simulink model "BLDC_speedcontroller_regenbraking"  (R2017a)
settings: Solver=VariableStepAuto  StartTime=0.0  StopTime=5  MaxStep=1e-4  RelTol=1e-3
undefined symbols (not defined in the file): Ion, Lithium, Ts
libraries: powerlib x14, simulink x12, electricdrivelib x2
settings Model: Creator=Jay Anil Puranik  LastModifiedBy=Jay Anil Puranik

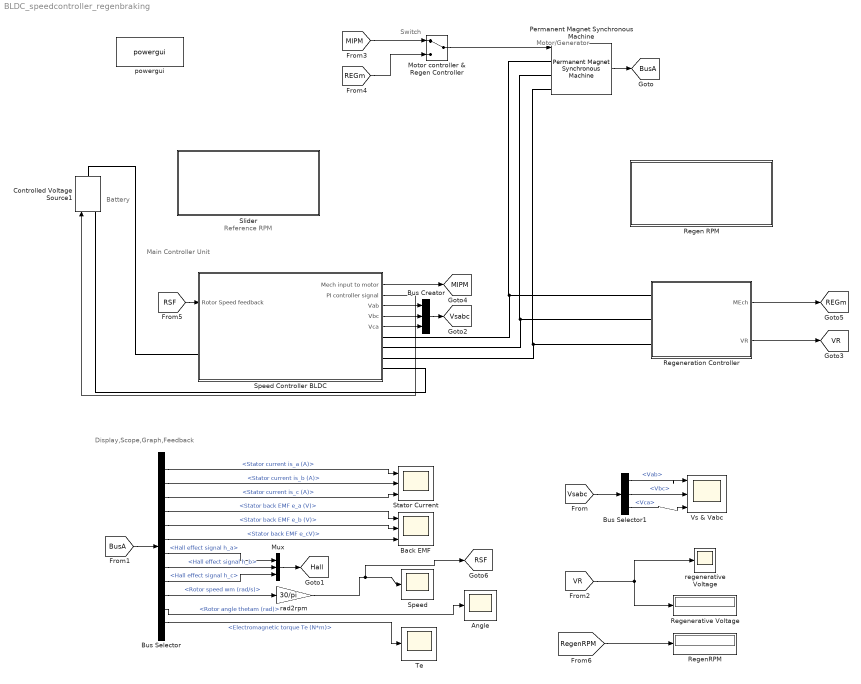
== system BLDC_speedcontroller_regenbraking ==
  note: Reference RPM
  note: Display,Scope,Graph,Feedback
  note: Main Controller Unit
  note: Motor/Generator
  note: Switch
  note: Battery
  " Angle " : Scope
  "Back EMF " : Scope  NumInputPorts=3
  Bus Creator : BusCreator  Inputs=3
  Bus Selector : BusSelector  OutputSignals=Stator current is_a (A),Stator current is_b (A),Stator current is_c (A),Stator back EMF e_a (V),Stator back EMF e_b (V),Stator back EMF e_cV),Hall effect signal h_a,Hall effect signal h_b,Hall effect signal h_c,Rotor speed wm (rad/s),Rotor angle thetam (rad),Electromagnetic torque Te (N*m)
  Bus Selector1 : BusSelector  OutputSignals=Vab,Vbc,Vca
  Controlled Voltage Source1 : powerlib/Electrical Sources/Controlled Voltage Source  Initialize=on  Source_Type=DC  Amplitude=110  Phase=0  Frequency=0  Measurements=Voltage
  "Motor controller & Regen Controller " : ManualSwitch
  Mux : Mux  Inputs=3
  Permanent Magnet Synchronous Machine : powerlib/Machines/Permanent Magnet Synchronous Machine  NbPhases=3  FluxDistribution=Trapezoidal  RotorType=Round  MechanicalLoad=Torque Tm  PresetModel=No  ShowDetailedParameters=on  MeasurementBus=off  Resistance=2.8750  Inductance=8.5e-3  dqInductances=[8.5e-3, 8.5e-3]  La=0.000835  MachineConstant=Flux linkage established by magnets (V.s)  Flux=0.175  VoltageCst=146.6077  TorqueCst=1.4  Flat=120  Mechanical=[ 0.8e-3, 1e-3 4]  PolePairs=4  InitialConditions=[0,0, 0,0]  InitialConditions5ph=[0 0 0 0 0 0]  TsPowergui=0  TsBlock=-1  RefAngle=90 degrees behind phase A axis (modified Park)
      settings: SourceProductName=Simscape Power Systems
  "Regen RPM " : Subsystem  DialogController=hmiCreateDDGDialog  IsWebBlock=on  mask(MWDashboardBlock){webBlockId=a570a540-91aa-4276-bd03-00008c0634f1, webBlockType=slider, ShowInLibBrowser=on, ShowInitialText=on, HMISrcModelName=BLDC_speedcontroller_regenbraking}
      mask prompts: webBlockId "WebBlock Id"; webBlockType "WebBlock Type"; HMISrcModelName "Source Model"
      mask help: SimulinkHMI:dialogs:SliderDialogDesc
      mask Help: helpview([docroot '/mapfiles/simulink.map'], 'hmi_slider')
      mask Display:
      | if strcmp(get_param(bdroot(gcb),'BlockDiagramType'), 'library')
      |     image([(matlabroot) '/toolbox/simulink/hmi/icons/Slider.png']);
      | end
  RegenRPM : Display
  Regeneration Controller : Subsystem
  Regenerative Voltage : Display
  Slider : Subsystem  DialogController=hmiCreateDDGDialog  IsWebBlock=on  mask(MWDashboardBlock){webBlockId=640ab695-851c-4546-9140-9b28d641b0e5, webBlockType=slider, ShowInLibBrowser=on, ShowInitialText=on, HMISrcModelName=BLDC_speedcontroller_regenbraking}
      mask prompts: webBlockId "WebBlock Id"; webBlockType "WebBlock Type"; HMISrcModelName "Source Model"
      mask help: SimulinkHMI:dialogs:SliderDialogDesc
      mask Help: helpview([docroot '/mapfiles/simulink.map'], 'hmi_slider')
      mask Display:
      | if strcmp(get_param(bdroot(gcb),'BlockDiagramType'), 'library')
      |     image([(matlabroot) '/toolbox/simulink/hmi/icons/Slider.png']);
      | end
  "Speed " : Scope
  Speed Controller BLDC : Subsystem
  "Stator Current " : Scope  NumInputPorts=3
  "Te " : Scope
  "Vs & Vabc " : Scope  NumInputPorts=3
  powergui : powerlib/powergui  Priority=2  SimulationMode=Continuous  SampleTime=Ts  frequency=60  Iterations=50  frequencyindice=0  Pbase=100e6  ErrMax=1e-4  UnitsV=kV  UnitsW=MW  buscounter=0  FunctionMessages=off  echomessages=off  EnableUseOfTLC=off  CurrentSourceSwitches=off  DisableSnubberDevices=off  DisableRonSwitches=off  DisableVfSwitches=off  DisplayEquations=off  SolverType=Tustin/Backward Euler (TBE)  Interpol=off  ExternalGateDelay=off  methode=off  Ts=100  x0status=blocks  SPID=on  SwTol=0  HookPort=off  RestoreLinks=warning  ResistiveCurrentMeasurement=off  Frange=[0:2:500]  Ylog=off  Xlog=on  ShowGrid=off  save=off  variable=ZData  structure=0  ZoomFFT=on  StartTime=0.0  cycles=1  DisplayStyle=1  fundamental=60  FreqAxis=off  MaxFrequency=1000  frequencyindicesteady=1  RmsSteady=1  display=off
  rad2rpm : Gain  Gain=30/pi
  regenerative Voltage : Scope
  tag scope: BusA=global, Hall=global, MIPM=global, REGm=global, RSF=global, VR=global, Vsabc=global
  wires:
  Bus Selector/1 -> "Stator Current "/1  "<Stator current is_a (A)>"
  Bus Selector/2 -> "Stator Current "/2  "<Stator current is_b (A)>"
  Bus Selector/3 -> "Stator Current "/3  "<Stator current is_c (A)>"
  Bus Selector/4 -> "Back EMF "/1  "<Stator back EMF e_a (V)>"
  Bus Selector/5 -> "Back EMF "/2  "<Stator back EMF e_b (V)>"
  Bus Selector/6 -> "Back EMF "/3  "<Stator back EMF e_cV)>"
  Bus Selector/7 -> Mux/1  "<Hall effect signal h_a>"
  Bus Selector/9 -> Mux/3  "<Hall effect signal h_c>"
  Bus Selector/8 -> Mux/2  "<Hall effect signal h_b>"
  Bus Selector/11 -> " Angle "/1  "<Rotor angle thetam (rad)>"
  Bus Selector/12 -> "Te "/1  "<Electromagnetic torque Te (N*m)>"
  Mux/1 -> [Hall]
  Permanent Magnet Synchronous Machine/1 -> [BusA]
  [Vsabc] -> Bus Selector1/1
  Bus Creator/1 -> [Vsabc]
  Speed Controller BLDC/3(Vab) -> Bus Creator/1
  Speed Controller BLDC/4(Vbc) -> Bus Creator/2
  Speed Controller BLDC/5(Vca) -> Bus Creator/3
  Bus Selector1/1 -> "Vs & Vabc "/1  "<Vab>"
  Bus Selector1/2 -> "Vs & Vabc "/2  "<Vbc>"
  Bus Selector1/3 -> "Vs & Vabc "/3  "<Vca>"
  [BusA] -> Bus Selector/1
  [VR] -> Regenerative Voltage/1, regenerative Voltage/1
  Speed Controller BLDC/1(Mech input to motor) -> [MIPM]
  Speed Controller BLDC/2(PI controller signal) -> Controlled Voltage Source1/1
  [MIPM] -> "Motor controller & Regen Controller "/1
  Regeneration Controller/2(VR) -> [VR]
  Regeneration Controller/1(MEch) -> [REGm]
  [REGm] -> "Motor controller & Regen Controller "/2
  [RSF] -> Speed Controller BLDC/1(Rotor Speed feedback)
  [RegenRPM] -> RegenRPM/1
  "Motor controller & Regen Controller "/1 -> Permanent Magnet Synchronous Machine/1
  Bus Selector/10 -> rad2rpm/1  "<Rotor speed wm (rad/s)>"
  rad2rpm/1 -> [RSF], "Speed "/1
  connections:
  Speed Controller BLDC/RConn1 -- Permanent Magnet Synchronous Machine/LConn1 -- Regeneration Controller/LConn1
  Speed Controller BLDC/RConn2 -- Regeneration Controller/LConn2 -- Permanent Magnet Synchronous Machine/LConn2
  Speed Controller BLDC/RConn3 -- Regeneration Controller/LConn3 -- Permanent Magnet Synchronous Machine/LConn3
  Speed Controller BLDC/LConn1 -- Controlled Voltage Source1/RConn1
  Speed Controller BLDC/RConn4 -- Controlled Voltage Source1/LConn1

== system BLDC_speedcontroller_regenbraking/Regen RPM  ==

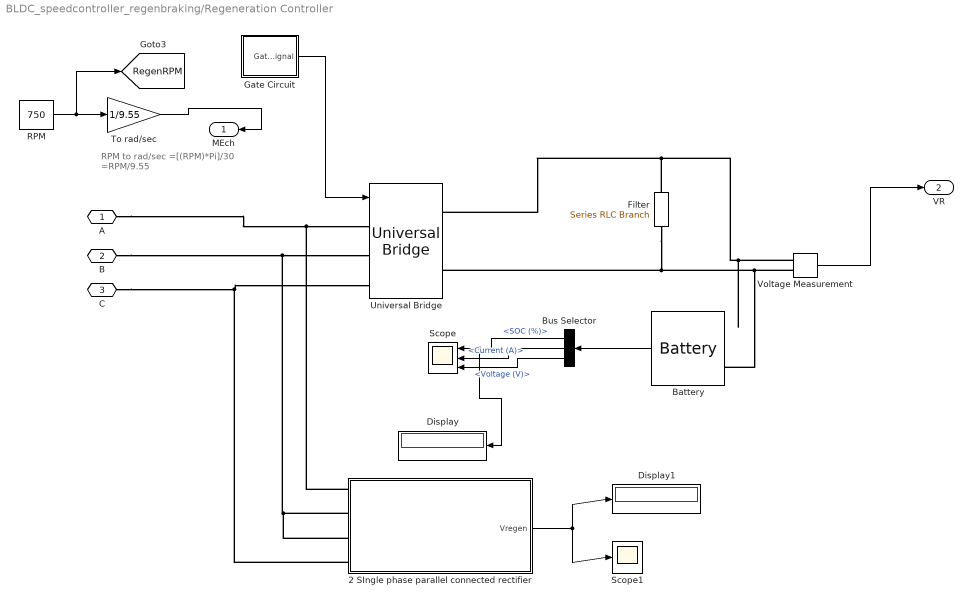
== system BLDC_speedcontroller_regenbraking/Regeneration Controller ==
  note: RPM to rad/sec
      | =[(RPM)*Pi]/30
      | =RPM/9.55
  "2 SIngle phase parallel connected rectifier " : Subsystem
  Battery : electricdrivelib/Extra Sources/Battery  BatType=Lithium-Ion  ShowTempParam=off  ThermalPreset=no  ShowAgeParam=off  NomV=7.2  NomQ=5.4  SOC=10  Batt_Tr=30  PresetModel=off  MaxQ=5.4  MinV=5.4  FullV=8.3807  Dis_rate=2.3478  R=0.013333  Normal_OP=4.8835  expZone="[7.7788      0.2653]"  current=[6.5 13 32.5]  Units=Time  Tci=20  NomT=20  T2=-30  MaxQ2=4.8  FullV2=7.1  Normal_OP2=5.655  expZone2="[6.58           1]"  Rca=0.6  ti=2000  Dp=0  Neq0=0  Tsim=1e6  Ta1=25  Qeol=5.4*0.9  Reol=0.013333*1.2  Char_age=[2.3478, 3]  Dis_age=[2.3478, 10]  N1=1500  N2=10500  N3=1000  N4=1400  Ta2=45  N5=950
  Bus Selector : BusSelector  OutputSignals=SOC (%),Current (A),Voltage (V)
  Display : Display
  Display1 : Display
  Filter : powerlib/Elements/Series RLC Branch  LConnTagsString=__new0  RConnTagsString=__new0  BranchType=C  Resistance=1  Inductance=1e-3  SetiL0=off  InitialCurrent=0  Capacitance=100e-6  Setx0=off  InitialVoltage=0  Measurements=None
  Gate Circuit : Subsystem
  "RPM " : Constant  Value=750
  Scope : Scope  NumInputPorts=3
  Scope1 : Scope
  To rad/sec : Gain  Gain=1/9.55
  Universal Bridge : powerlib/Power Electronics/Universal Bridge  Arms=3  SnubberResistance=1e5  SnubberCapacitance=inf  Device=Thyristors  Ron=1e-3  Lon=0  ForwardVoltages="[  0  0  ]"  ForwardVoltage=0  GTOparameters=[ 10e-6 , 20e-6 ]  IGBTparameters=[ 1e-6 , 2e-6 ]  Measurements=None  Measurements_2=None  converterType=Rectifier
  Voltage Measurement : powerlib/Measurements/Voltage Measurement  PhasorSimulation=off  OutputType=Magnitude  PSBequivalent=0
  A : PMIOPort  Port=1  Side=Left
  B : PMIOPort  Port=2  Side=Left
  C : PMIOPort  Port=3  Side=Left
  MEch : Outport
  VR : Outport  Port=2
  tag scope: RegenRPM=global
  wires:
  Gate Circuit/1("Gate Signal ") -> Universal Bridge/1
  Voltage Measurement/1 -> VR/1
  To rad/sec/1 -> MEch/1
  "RPM "/1 -> [RegenRPM], To rad/sec/1
  Battery/1 -> Bus Selector/1
  Bus Selector/1 -> Display/1, Scope/1  "<SOC (%)>"
  Bus Selector/2 -> Scope/2  "<Current (A)>"
  Bus Selector/3 -> Scope/3  "<Voltage (V)>"
  "2 SIngle phase parallel connected rectifier "/1("Vregen ") -> Display1/1, Scope1/1
  connections:
  B/RConn1 -- "2 SIngle phase parallel connected rectifier "/LConn3 -- "2 SIngle phase parallel connected rectifier "/LConn2 -- Universal Bridge/LConn2
  A/RConn1 -- "2 SIngle phase parallel connected rectifier "/LConn1 -- Universal Bridge/LConn1
  C/RConn1 -- "2 SIngle phase parallel connected rectifier "/LConn4 -- Universal Bridge/LConn3
  Voltage Measurement/LConn2 -- Battery/LConn2 -- Universal Bridge/RConn2 -- Filter/RConn1
  Voltage Measurement/LConn1 -- Filter/LConn1 -- Universal Bridge/RConn1

== system BLDC_speedcontroller_regenbraking/Slider ==

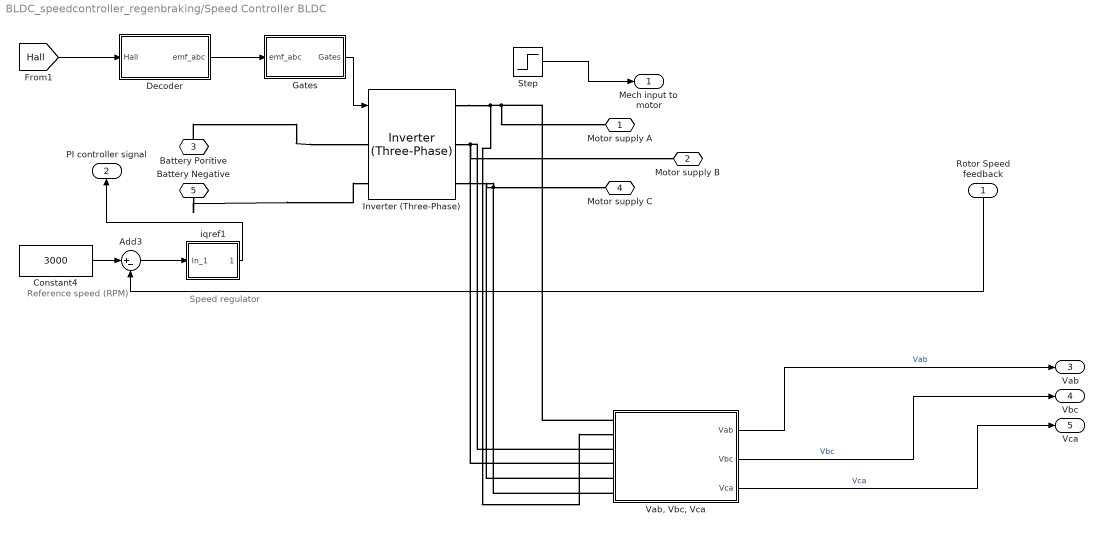
== system BLDC_speedcontroller_regenbraking/Speed Controller BLDC ==
  note: Speed
      | regulator
  note: Reference
      | speed (RPM)
  Rotor Speed feedback : Inport
  Add3 : Sum  Inputs=|+-
  Constant4 : Constant  Value=3000
  Decoder : Subsystem
  Gates : Subsystem
  Inverter (Three-Phase) : electricdrivelib/Fundamental Drive Blocks/Inverter (Three-Phase)  OverrideUsingVariant=Detailed  detailLevel=Detailed  driveType=Field-oriented control  Ts=2e-6  SnubberResistance=500  SnubberCapacitance=inf  Device=IGBT / Diodes  Ron=1  ForwardVoltages=[1.2,1.2]  GTOparameters=[1e-6,2e-6]  IGBTparameters=[1e-6,2e-6]  Measurements=All voltages and currents  converterType=Inverter  SourceFrequency=0  ReferenceFrame=Rotor  dqInductances=[8.5e-3,8.5e-3]  Inductance=8.5e-3  Ls=0  Resistance=0.2  Flux=0  Stator_sm=[2.01e-3,4.289e-4,4.477e-3,1.354e-3]  Stator_im=[14.85e-3,0.3027e-3]  Rotor=[9.295e-3,0.3027e-3]  Lm=10.46e-3  p=4
      settings: AttributesFormatString=%<BlockChoice>  SourceProductName=Simscape Power Systems  SourceProductBaseCode=PS
  Step : Step  Time=.1  After=3  SampleTime=0
  "Vab, Vbc, Vca" : Subsystem
  iqref1 : Subsystem  mask(PI Controller){I=16.61, P=.013, sat=[-100, 100]}
      mask prompts: I "Integral"; P "Proportional:"; sat "Minimum and maximum outputs:"
      mask init:
      | min=sat(1);max=sat(2);
      mask Display: disp('PI')
  Motor supply A : PMIOPort  Port=1  Side=Right
  Motor supply B : PMIOPort  Port=2  Side=Right
  "Battery Poritive " : PMIOPort  Port=3  Side=Left
  Motor supply C : PMIOPort  Port=4  Side=Right
  Battery Negative : PMIOPort  Port=5  Side=Right
  Mech input to motor : Outport
  PI controller signal : Outport  Port=2
  Vab : Outport  Port=3
  Vbc : Outport  Port=4
  Vca : Outport  Port=5
  wires:
  Rotor Speed feedback/1 -> Add3/2
  [Hall] -> Decoder/1("Hall ")
  Step/1 -> Mech input to motor/1
  Gates/1(Gates) -> Inverter (Three-Phase)/1
  Add3/1 -> iqref1/1(In_1)
  Constant4/1 -> Add3/1
  Decoder/1(emf_abc) -> Gates/1("emf_abc ")
  "Vab, Vbc, Vca"/3("Vca ") -> Vca/1  "Vca"
  "Vab, Vbc, Vca"/1("Vab ") -> Vab/1  "Vab"
  "Vab, Vbc, Vca"/2("Vbc ") -> Vbc/1  "Vbc"
  iqref1/1(Out_1) -> PI controller signal/1
  connections:
  "Vab, Vbc, Vca"/LConn1 -- Inverter (Three-Phase)/RConn1 -- "Vab, Vbc, Vca"/LConn2 -- Motor supply A/RConn1
  Battery Negative/RConn1 -- Inverter (Three-Phase)/LConn2
  "Battery Poritive "/RConn1 -- Inverter (Three-Phase)/LConn1
  Inverter (Three-Phase)/RConn2 -- "Vab, Vbc, Vca"/LConn3 -- Motor supply B/RConn1 -- "Vab, Vbc, Vca"/LConn4
  "Vab, Vbc, Vca"/LConn6 -- "Vab, Vbc, Vca"/LConn5 -- Inverter (Three-Phase)/RConn3 -- Motor supply C/RConn1

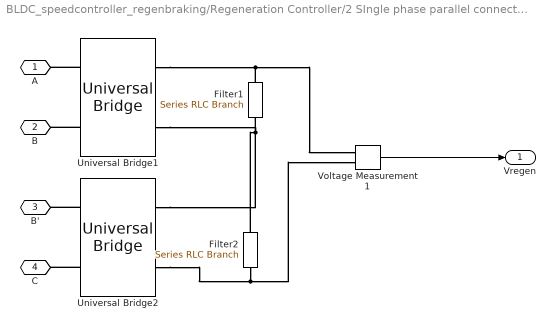
== system BLDC_speedcontroller_regenbraking/Regeneration Controller/2 SIngle phase parallel connected rectifier  ==
  Filter1 : powerlib/Elements/Series RLC Branch  LConnTagsString=__new0  RConnTagsString=__new0  BranchType=C  Resistance=1  Inductance=1e-3  SetiL0=off  InitialCurrent=0  Capacitance=100e-6  Setx0=off  InitialVoltage=0  Measurements=None
  Filter2 : powerlib/Elements/Series RLC Branch  LConnTagsString=__new0  RConnTagsString=__new0  BranchType=C  Resistance=1  Inductance=1e-3  SetiL0=off  InitialCurrent=0  Capacitance=100e-6  Setx0=off  InitialVoltage=0  Measurements=None
  Universal Bridge1 : powerlib/Power Electronics/Universal Bridge  Arms=2  SnubberResistance=1e5  SnubberCapacitance=inf  Device=Diodes  Ron=1e-3  Lon=0  ForwardVoltages="[  0  0  ]"  ForwardVoltage=0  GTOparameters=[ 10e-6 , 20e-6 ]  IGBTparameters=[ 1e-6 , 2e-6 ]  Measurements=None  Measurements_2=None  converterType=Rectifier
  Universal Bridge2 : powerlib/Power Electronics/Universal Bridge  Arms=2  SnubberResistance=1e5  SnubberCapacitance=inf  Device=Diodes  Ron=1e-3  Lon=0  ForwardVoltages="[  0  0  ]"  ForwardVoltage=0  GTOparameters=[ 10e-6 , 20e-6 ]  IGBTparameters=[ 1e-6 , 2e-6 ]  Measurements=None  Measurements_2=None  converterType=Rectifier
  Voltage Measurement1 : powerlib/Measurements/Voltage Measurement  PhasorSimulation=off  OutputType=Magnitude  PSBequivalent=0
  A : PMIOPort  Port=1  Side=Left
  B : PMIOPort  Port=2  Side=Left
  B' : PMIOPort  Port=3  Side=Left
  C : PMIOPort  Port=4  Side=Left
  "Vregen " : Outport
  wires:
  Voltage Measurement1/1 -> "Vregen "/1
  connections:
  Universal Bridge2/LConn1 -- B'/RConn1
  Universal Bridge1/LConn2 -- B/RConn1
  Universal Bridge1/LConn1 -- A/RConn1
  Universal Bridge2/LConn2 -- C/RConn1
  Universal Bridge1/RConn2 -- Filter2/LConn1 -- Universal Bridge2/RConn1 -- Filter1/RConn1
  Universal Bridge2/RConn2 -- Voltage Measurement1/LConn2 -- Filter2/RConn1
  Universal Bridge1/RConn1 -- Voltage Measurement1/LConn1 -- Filter1/LConn1

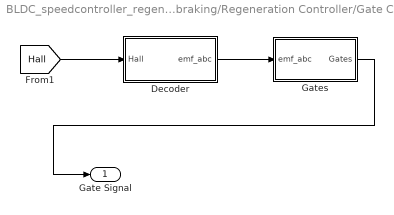
== system BLDC_speedcontroller_regenbraking/Regeneration Controller/Gate Circuit ==
  Decoder : Subsystem
  Gates : Subsystem
  "Gate Signal " : Outport
  wires:
  [Hall] -> Decoder/1("Hall ")
  Decoder/1(emf_abc) -> Gates/1("emf_abc ")
  Gates/1(Gates) -> "Gate Signal "/1

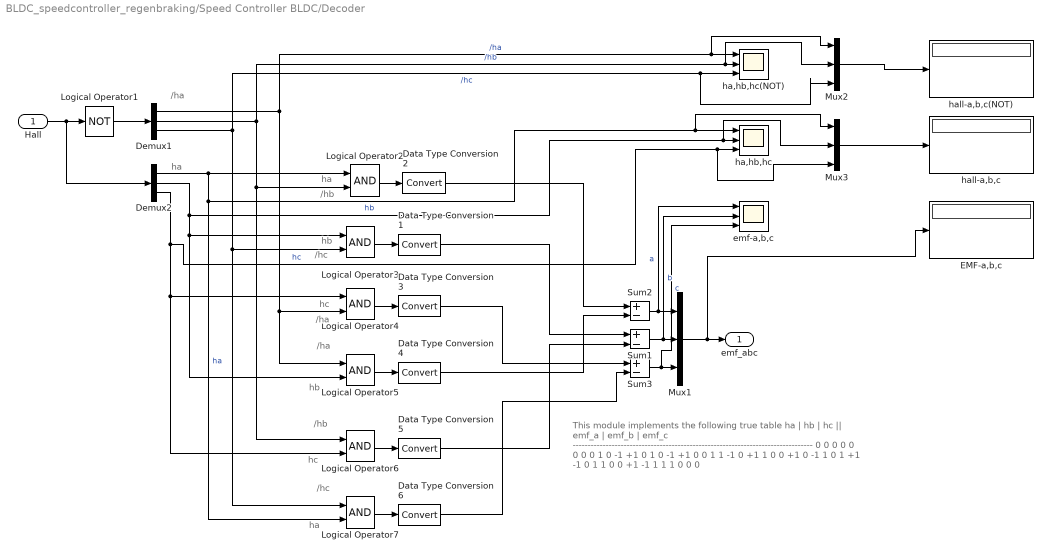
== system BLDC_speedcontroller_regenbraking/Speed Controller BLDC/Decoder ==
  note: /ha
  note: ha
  note: ha
  note: /hb
  note: hb
  note: /hc
  note: hc
  note: /ha
  note: /ha
  note: hb
  note: /hb
  note: hc
  note: /hc
  note: ha
  note: This module implements the following true table
      |
      |    ha   |   hb   |   hc   ||   emf_a   |   emf_b   |   emf_c
      |     --------------------------------------------------------------------------------
      | 0          0         0          0               0               0
      | 0          0         1          0               -1              +1
      | 0          1         0          -1              +1                0
      | 0          1         1          -1               0               +1
      | 1          0         0         +1               0               -1
      | 1          0         1         +1              -1                0
      | 1          1         0          0              +1               -1
      | 1          1         1          0               0                0
  "Hall " : Inport
  Data Type Conversion{1..6} (6 alike) : DataTypeConversion
  Demux1 : Demux  Outputs=3
  Demux2 : Demux  Outputs=3
  EMF-a,b,c : Display
  Logical Operator1 : Logic  Operator=NOT  AllPortsSameDT=off  OutDataTypeStr=boolean
  Logical Operator{2..7} (6 alike) : Logic  AllPortsSameDT=off  OutDataTypeStr=boolean
  Mux1 : Mux  Inputs=3
  Mux2 : Mux  Inputs=3
  Mux3 : Mux  Inputs=3
  Sum1 : Sum  Inputs=+-  OutDataTypeStr=double
  Sum2 : Sum  Inputs=+-  OutDataTypeStr=double
  Sum3 : Sum  Inputs=+-  OutDataTypeStr=double
  emf-a,b,c : Scope  NumInputPorts=3
  ha,hb,hc : Scope  NumInputPorts=3
  ha,hb,hc(NOT) : Scope  NumInputPorts=3
  hall-a,b,c : Display
  hall-a,b,c(NOT) : Display
  emf_abc : Outport
  wires:
  "Hall "/1 -> Logical Operator1/1, Demux2/1
  Logical Operator1/1 -> Demux1/1
  Demux2/3 -> Mux3/3, ha,hb,hc/3, Logical Operator4/1, Logical Operator6/2  "hc"
  Demux2/2 -> Mux3/2, ha,hb,hc/2, Logical Operator3/1, Logical Operator5/2  "hb"
  Demux1/3 -> Logical Operator3/2, Logical Operator7/1, Mux2/3, ha,hb,hc(NOT)/3  "/hc"
  Demux1/2 -> Logical Operator2/2, Logical Operator6/1, Mux2/2, ha,hb,hc(NOT)/2  "/hb"
  Demux1/1 -> Logical Operator4/2, Logical Operator5/1, Mux2/1, ha,hb,hc(NOT)/1  "/ha"
  Logical Operator2/1 -> Data Type Conversion2/1
  Sum2/1 -> emf-a,b,c/1, Mux1/1  "a"
  Sum1/1 -> emf-a,b,c/2, Mux1/2  "b"
  Sum3/1 -> emf-a,b,c/3, Mux1/3  "c"
  Mux1/1 -> EMF-a,b,c/1, emf_abc/1
  Logical Operator3/1 -> Data Type Conversion1/1
  Logical Operator4/1 -> Data Type Conversion3/1
  Logical Operator5/1 -> Data Type Conversion4/1
  Logical Operator6/1 -> Data Type Conversion5/1
  Logical Operator7/1 -> Data Type Conversion6/1
  Data Type Conversion2/1 -> Sum2/1
  Data Type Conversion4/1 -> Sum2/2
  Data Type Conversion1/1 -> Sum1/1
  Data Type Conversion5/1 -> Sum1/2
  Data Type Conversion3/1 -> Sum3/1
  Data Type Conversion6/1 -> Sum3/2
  Demux2/1 -> Logical Operator2/1, Mux3/1, ha,hb,hc/1, Logical Operator7/2  "ha"
  Mux3/1 -> hall-a,b,c/1
  Mux2/1 -> hall-a,b,c(NOT)/1

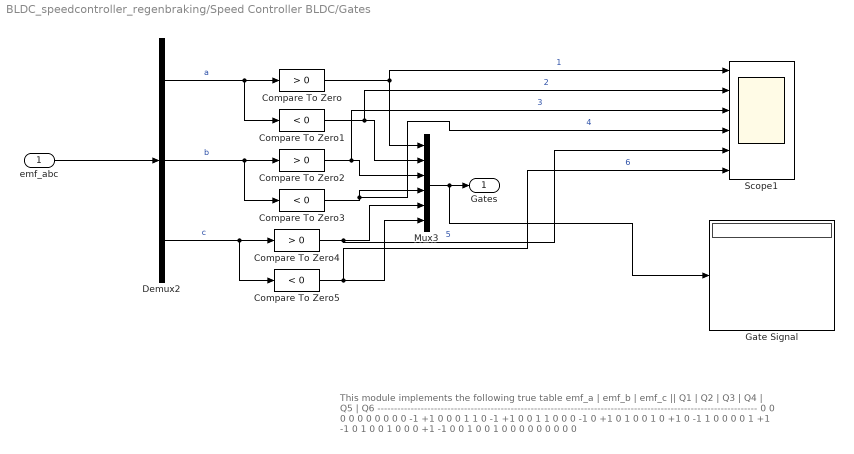
== system BLDC_speedcontroller_regenbraking/Speed Controller BLDC/Gates ==
  note: This module implements the following true table
      |
      |    emf_a   |   emf_b   |   emf_c   ||   Q1   |   Q2   |   Q3   |   Q4   |   Q5   |   Q6
      |     ------------------------------------------------------------------------------------------------------------------
      |       0              0                0            0          0          0           0        0        0
      |       0               -1              +1          0          0          0           1        1        0
      |     -1              +1                0          0          1          1           0        0        0
      |     -1               0               +1          0          1         0           0        1        0
      |    +1               0                -1          1          0          0           0        0        1
      |    +1              -1                0           1          0          0           1        0        0
      |      0              +1               -1           0          0          1           0        0        1
      |     0              0                0             0          0          0           0        0        0
  "emf_abc " : Inport
  Compare To Zero : simulink/Logic and Bit Operations/Compare To Zero  relop=>  OutDataTypeStr=boolean  ZeroCross=off
  Compare To Zero1 : simulink/Logic and Bit Operations/Compare To Zero  relop=<  OutDataTypeStr=boolean  ZeroCross=off
  Compare To Zero2 : simulink/Logic and Bit Operations/Compare To Zero  relop=>  OutDataTypeStr=boolean  ZeroCross=off
  Compare To Zero3 : simulink/Logic and Bit Operations/Compare To Zero  relop=<  OutDataTypeStr=boolean  ZeroCross=off
  Compare To Zero4 : simulink/Logic and Bit Operations/Compare To Zero  relop=>  OutDataTypeStr=boolean  ZeroCross=off
  Compare To Zero5 : simulink/Logic and Bit Operations/Compare To Zero  relop=<  OutDataTypeStr=boolean  ZeroCross=off
  Demux2 : Demux  Outputs=3
  Gate Signal : Display
  Mux3 : Mux  Inputs=6
  Scope1 : Scope  NumInputPorts=6
  Gates : Outport
  wires:
  "emf_abc "/1 -> Demux2/1
  Mux3/1 -> Gate Signal/1, Gates/1
  Demux2/1 -> Compare To Zero/1, Compare To Zero1/1  "a"
  Demux2/2 -> Compare To Zero2/1, Compare To Zero3/1  "b"
  Demux2/3 -> Compare To Zero4/1, Compare To Zero5/1  "c"
  Compare To Zero/1 -> Scope1/1, Mux3/1  "1"
  Compare To Zero1/1 -> Scope1/2, Mux3/2  "2"
  Compare To Zero2/1 -> Scope1/3, Mux3/3  "3"
  Compare To Zero3/1 -> Scope1/4, Mux3/4  "4"
  Compare To Zero5/1 -> Scope1/6, Mux3/6  "6"
  Compare To Zero4/1 -> Scope1/5, Mux3/5  "5"

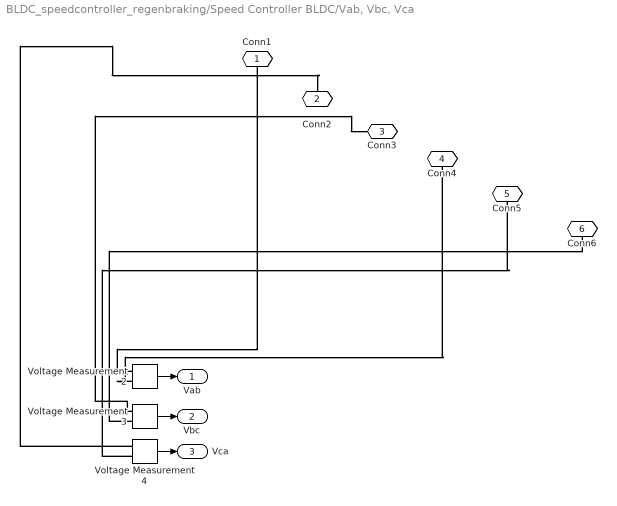
== system BLDC_speedcontroller_regenbraking/Speed Controller BLDC/Vab, Vbc, Vca ==
  Voltage Measurement2 : powerlib/Measurements/Voltage Measurement  PhasorSimulation=off  OutputType=Complex  PSBequivalent=0
  Voltage Measurement3 : powerlib/Measurements/Voltage Measurement  PhasorSimulation=off  OutputType=Complex  PSBequivalent=0
  Voltage Measurement4 : powerlib/Measurements/Voltage Measurement  PhasorSimulation=off  OutputType=Complex  PSBequivalent=0
  Conn1 : PMIOPort  Port=1  Side=Left
  Conn2 : PMIOPort  Port=2  Side=Left
  Conn3 : PMIOPort  Port=3  Side=Left
  Conn4 : PMIOPort  Port=4  Side=Left
  Conn5 : PMIOPort  Port=5  Side=Left
  Conn6 : PMIOPort  Port=6  Side=Left
  "Vab " : Outport
  "Vbc " : Outport  Port=2
  "Vca " : Outport  Port=3
  wires:
  Voltage Measurement2/1 -> "Vab "/1
  Voltage Measurement4/1 -> "Vca "/1
  Voltage Measurement3/1 -> "Vbc "/1
  connections:
  Voltage Measurement3/LConn2 -- Conn6/RConn1
  Voltage Measurement4/LConn1 -- Conn2/RConn1
  Voltage Measurement4/LConn2 -- Conn5/RConn1
  Voltage Measurement3/LConn1 -- Conn3/RConn1
  Voltage Measurement2/LConn1 -- Conn1/RConn1
  Voltage Measurement2/LConn2 -- Conn4/RConn1

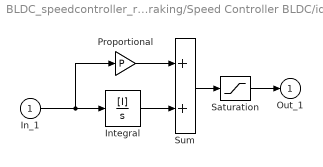
== system BLDC_speedcontroller_regenbraking/Speed Controller BLDC/iqref1 ==
  In_1 : Inport
  Integral : TransferFcn  Numerator=[I]  Denominator=[1 0]
  Proportional : Gain  Gain=P  SaturateOnIntegerOverflow=on  OutDataTypeStr=Inherit: Same as input  ParamDataTypeStr=Inherit: Same as input
  Saturation : Saturate  UpperLimit=max  LowerLimit=min
  Sum : Sum  SaturateOnIntegerOverflow=on  InputSameDT=on  OutDataTypeStr=Inherit: Same as first input
  Out_1 : Outport  InitialOutput=0
  wires:
  Saturation/1 -> Out_1/1
  Sum/1 -> Saturation/1
  Proportional/1 -> Sum/1
  In_1/1 -> Proportional/1, Integral/1
  Integral/1 -> Sum/2

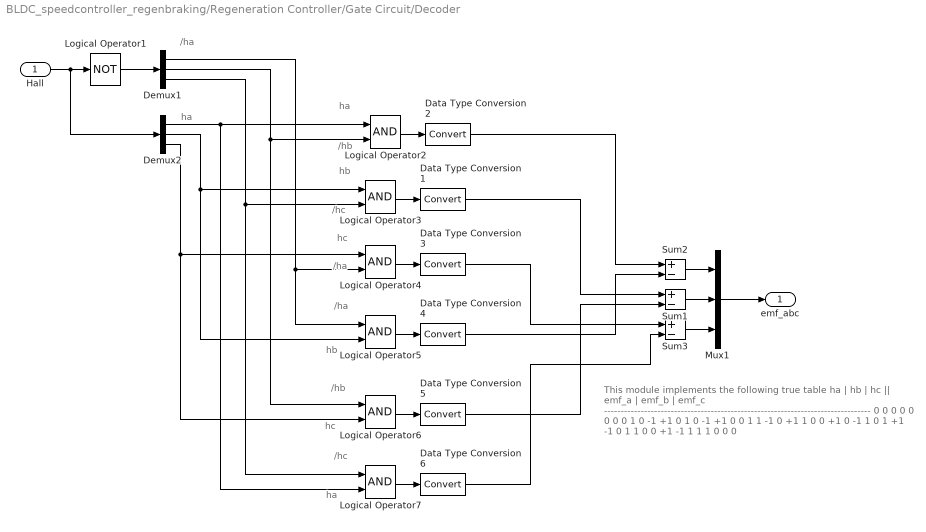
== system BLDC_speedcontroller_regenbraking/Regeneration Controller/Gate Circuit/Decoder ==
  note: /ha
  note: ha
  note: ha
  note: /hb
  note: hb
  note: /hc
  note: hc
  note: /ha
  note: /ha
  note: hb
  note: /hb
  note: hc
  note: /hc
  note: ha
  note: This module implements the following true table
      |
      |    ha   |   hb   |   hc   ||   emf_a   |   emf_b   |   emf_c
      |     --------------------------------------------------------------------------------
      | 0          0         0          0               0               0
      | 0          0         1          0               -1              +1
      | 0          1         0          -1              +1                0
      | 0          1         1          -1               0               +1
      | 1          0         0         +1               0               -1
      | 1          0         1         +1              -1                0
      | 1          1         0          0              +1               -1
      | 1          1         1          0               0                0
  "Hall " : Inport
  Data Type Conversion{1..6} (6 alike) : DataTypeConversion
  Demux1 : Demux  Outputs=3
  Demux2 : Demux  Outputs=3
  Logical Operator1 : Logic  Operator=NOT  AllPortsSameDT=off  OutDataTypeStr=boolean
  Logical Operator{2..7} (6 alike) : Logic  AllPortsSameDT=off  OutDataTypeStr=boolean
  Mux1 : Mux  Inputs=3
  Sum1 : Sum  Inputs=+-  OutDataTypeStr=double
  Sum2 : Sum  Inputs=+-  OutDataTypeStr=double
  Sum3 : Sum  Inputs=+-  OutDataTypeStr=double
  emf_abc : Outport
  wires:
  "Hall "/1 -> Logical Operator1/1, Demux2/1
  Logical Operator1/1 -> Demux1/1
  Demux2/3 -> Logical Operator4/1, Logical Operator6/2
  Demux2/2 -> Logical Operator3/1, Logical Operator5/2
  Demux2/1 -> Logical Operator2/1, Logical Operator7/2
  Demux1/3 -> Logical Operator3/2, Logical Operator7/1
  Demux1/2 -> Logical Operator2/2, Logical Operator6/1
  Demux1/1 -> Logical Operator4/2, Logical Operator5/1
  Logical Operator2/1 -> Data Type Conversion2/1
  Sum2/1 -> Mux1/1
  Sum1/1 -> Mux1/2
  Sum3/1 -> Mux1/3
  Mux1/1 -> emf_abc/1
  Logical Operator3/1 -> Data Type Conversion1/1
  Logical Operator4/1 -> Data Type Conversion3/1
  Logical Operator5/1 -> Data Type Conversion4/1
  Logical Operator6/1 -> Data Type Conversion5/1
  Logical Operator7/1 -> Data Type Conversion6/1
  Data Type Conversion2/1 -> Sum2/1
  Data Type Conversion4/1 -> Sum2/2
  Data Type Conversion1/1 -> Sum1/1
  Data Type Conversion5/1 -> Sum1/2
  Data Type Conversion3/1 -> Sum3/1
  Data Type Conversion6/1 -> Sum3/2

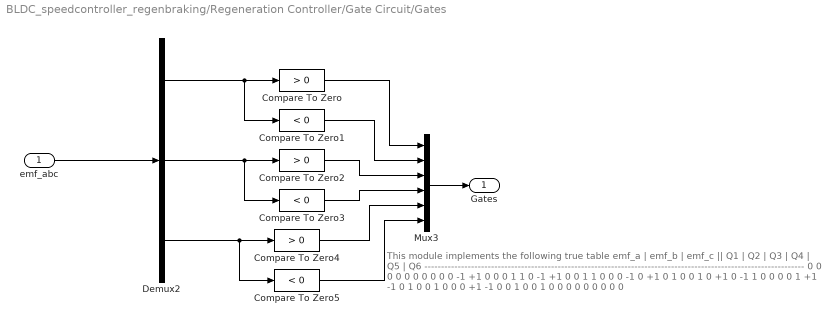
== system BLDC_speedcontroller_regenbraking/Regeneration Controller/Gate Circuit/Gates ==
  note: This module implements the following true table
      |
      |    emf_a   |   emf_b   |   emf_c   ||   Q1   |   Q2   |   Q3   |   Q4   |   Q5   |   Q6
      |     ------------------------------------------------------------------------------------------------------------------
      |       0              0                0            0          0          0           0        0        0
      |       0               -1              +1          0          0          0           1        1        0
      |     -1              +1                0          0          1          1           0        0        0
      |     -1               0               +1          0          1         0           0        1        0
      |    +1               0                -1          1          0          0           0        0        1
      |    +1              -1                0           1          0          0           1        0        0
      |      0              +1               -1           0          0          1           0        0        1
      |     0              0                0             0          0          0           0        0        0
  "emf_abc " : Inport
  Compare To Zero : simulink/Logic and Bit Operations/Compare To Zero  relop=>  OutDataTypeStr=boolean  ZeroCross=off
  Compare To Zero1 : simulink/Logic and Bit Operations/Compare To Zero  relop=<  OutDataTypeStr=boolean  ZeroCross=off
  Compare To Zero2 : simulink/Logic and Bit Operations/Compare To Zero  relop=>  OutDataTypeStr=boolean  ZeroCross=off
  Compare To Zero3 : simulink/Logic and Bit Operations/Compare To Zero  relop=<  OutDataTypeStr=boolean  ZeroCross=off
  Compare To Zero4 : simulink/Logic and Bit Operations/Compare To Zero  relop=>  OutDataTypeStr=boolean  ZeroCross=off
  Compare To Zero5 : simulink/Logic and Bit Operations/Compare To Zero  relop=<  OutDataTypeStr=boolean  ZeroCross=off
  Demux2 : Demux  Outputs=3
  Mux3 : Mux  Inputs=6
  Gates : Outport
  wires:
  "emf_abc "/1 -> Demux2/1
  Mux3/1 -> Gates/1
  Demux2/1 -> Compare To Zero/1, Compare To Zero1/1
  Demux2/2 -> Compare To Zero2/1, Compare To Zero3/1
  Demux2/3 -> Compare To Zero4/1, Compare To Zero5/1
  Compare To Zero/1 -> Mux3/1
  Compare To Zero1/1 -> Mux3/2
  Compare To Zero2/1 -> Mux3/3
  Compare To Zero3/1 -> Mux3/4
  Compare To Zero4/1 -> Mux3/5
  Compare To Zero5/1 -> Mux3/6
